simulink model "LC0419_nicholasye_fft"  (R2021b)
settings: Solver=VariableStepAuto  StartTime=0.0  StopTime=0.4  MaxStep=1e-4  RelTol=1e-3
libraries: spsSeriesRLCBranchLib x5, spsCurrentMeasurementLib x2, spsVoltageMeasurementLib x2, spsControlledVoltageSourceLib x1, spsGroundLib x1, spsTriangleGeneratorLib x1, spspowerguiLib x1
settings Model: Creator=98038  LastModifiedBy=NicholasYe
settings SolverCC: AlgebraicLoopSolver=TrustRegion
settings DataIOCC: ReturnWorkspaceOutputs=off
settings DebuggingCC: SFMachineParentedDataDiag=warning  ArithmeticOperatorsInVariantConditions=warning
settings SFSimCC: SimUseLocalCustomCode=off  CustomCodeUndefinedFunction=UseInterfaceOnly
settings RTWCC: RTWUseLocalCustomCode=off

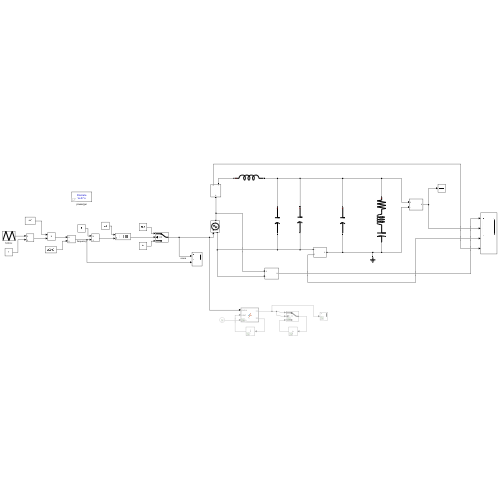
[thumbnail: Simulink's stored preview of the top-level diagram]
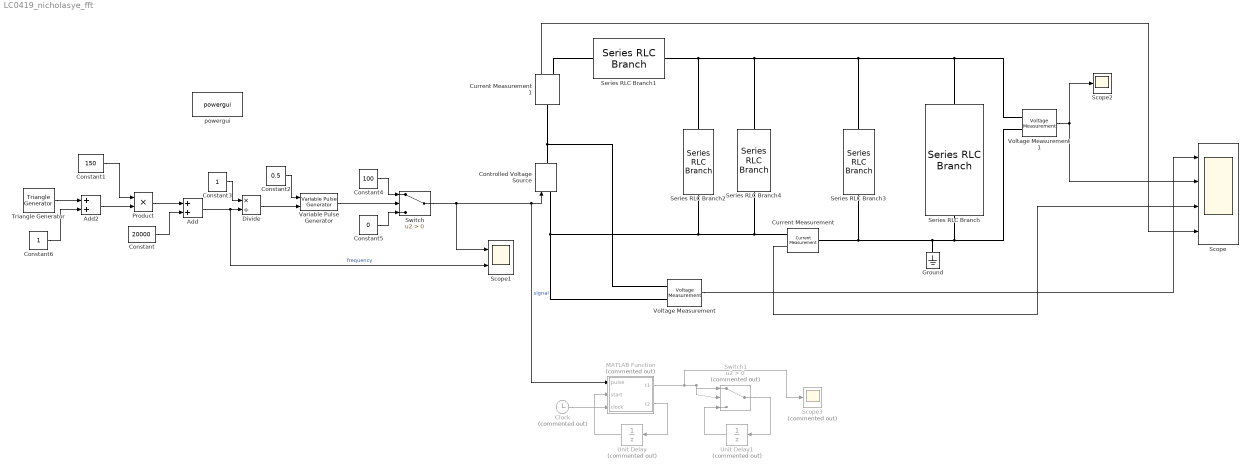
== system LC0419_nicholasye_fft ==
  Add : Sum
  Add2 : Sum
  Clock : Clock  Commented=on
  Constant : Constant  Value=20000
  Constant1 : Constant  Value=150
  Constant2 : Constant  Value=0.5
  Constant3 : Constant
  Constant4 : Constant  Value=100
  Constant5 : Constant  Value=0
  Constant6 : Constant
  Controlled Voltage Source : spsControlledVoltageSourceLib/Controlled Voltage Source  Initialize=off  Source_Type=AC  Amplitude=1  Phase=0  Frequency=20000  Measurements=Voltage
  Current Measurement : spsCurrentMeasurementLib/Current Measurement  PhasorSimulation=off  OutputType=Complex  PSBequivalent=0
  Current Measurement1 : spsCurrentMeasurementLib/Current Measurement  PhasorSimulation=off  OutputType=Complex  PSBequivalent=0
  Divide : Product  Inputs=*/
  Ground : spsGroundLib/Ground  LConnTagsString=a
  MATLAB Function : MATLAB Function  Commented=on  TreatAsAtomicUnit=on
  Product : Product
  Scope : Scope  NumInputPorts=4
  Scope1 : Scope  NumInputPorts=2
  Scope2 : Scope
  Scope3 : Scope  Commented=on
  Series RLC Branch : spsSeriesRLCBranchLib/Series RLC Branch  LConnTagsString=__new0  RConnTagsString=__new0  BranchType=RLC  Resistance=124.09  Inductance=1.463  SetiL0=off  InitialCurrent=0  Capacitance=42.528e-12  Setx0=off  InitialVoltage=0  Measurements=None
  Series RLC Branch1 : spsSeriesRLCBranchLib/Series RLC Branch  LConnTagsString=__new0  RConnTagsString=__new0  BranchType=L  Resistance=0  Inductance=0.00134  SetiL0=off  InitialCurrent=0  Capacitance=inf  Setx0=off  InitialVoltage=0  Measurements=None
  Series RLC Branch2 : spsSeriesRLCBranchLib/Series RLC Branch  LConnTagsString=__new0  RConnTagsString=__new0  BranchType=C  Resistance=0  Inductance=inf  SetiL0=off  InitialCurrent=0  Capacitance=6.8e-9  Setx0=off  InitialVoltage=0  Measurements=None
  Series RLC Branch3 : spsSeriesRLCBranchLib/Series RLC Branch  LConnTagsString=__new0  RConnTagsString=__new0  BranchType=C  Resistance=0  Inductance=inf  SetiL0=off  InitialCurrent=0  Capacitance=12.023e-9  Setx0=off  InitialVoltage=0  Measurements=None
  Series RLC Branch4 : spsSeriesRLCBranchLib/Series RLC Branch  LConnTagsString=__new0  RConnTagsString=__new0  BranchType=C  Resistance=0  Inductance=inf  SetiL0=off  InitialCurrent=0  Capacitance=6.8e-9  Setx0=off  InitialVoltage=0  Measurements=None
  Switch : Switch  Criteria=u2 > Threshold
  Switch1 : Switch  Commented=on  Criteria=u2 > Threshold
  Triangle Generator : spsTriangleGeneratorLib/Triangle Generator  Freq=500  Phase=0  Ts=0
      settings: AttributesFormatString=%<Freq>Hz
  Unit Delay : UnitDelay  Commented=on  SampleTime=-1  HasFrameUpgradeWarning=on
  Unit Delay1 : UnitDelay  Commented=on  SampleTime=-1  HasFrameUpgradeWarning=on
  Variable Pulse Generator : VariablePulseGenerator  SampleTime=0.1
  Voltage Measurement : spsVoltageMeasurementLib/Voltage Measurement  PhasorSimulation=off  OutputType=Complex  PSBequivalent=0
  Voltage Measurement1 : spsVoltageMeasurementLib/Voltage Measurement  PhasorSimulation=off  OutputType=Complex  PSBequivalent=0
  powergui : spspowerguiLib/powergui  Priority=1  SimulationMode=Discrete  SampleTime=1e-7  frequency=60  Iterations=50  frequencyindice=0  Pbase=100e6  ErrMax=1e-4  UnitsV=kV  UnitsW=MW  buscounter=0  FunctionMessages=off  echomessages=off  EnableUseOfTLC=off  CurrentSourceSwitches=off  DisableSnubberDevices=off  DisableRonSwitches=off  DisableVfSwitches=off  DisplayEquations=off  AutomaticDiscreteSolvers=off  SolverType=Tustin/Backward Euler (TBE)  Interpol=off  ExternalGateDelay=off  methode=off  Ts=100  x0status=blocks  SPID=on  SwTol=0  HookPort=off  NonlinearTolerance=1e-4  nMaxIteration=100  ContinueOnMaxIteration=off  RestoreLinks=warning  ResistiveCurrentMeasurement=off  Frange=[0:2:500]  Ylog=off  Xlog=on  ShowGrid=off  save=off  variable=ZData  structure=0  ZoomFFT=off  StartTime=0.0  cycles=1  DisplayStyle=1  fundamental=60  FreqAxis=off  MaxFrequency=1000  frequencyindicesteady=1  RmsSteady=1  display=off
  wires:
  Constant/1 -> Add/2
  Add2/1 -> Product/2
  Constant6/1 -> Add2/2
  Triangle Generator/1 -> Add2/1
  Constant3/1 -> Divide/1
  Constant2/1 -> Variable Pulse Generator/1
  Add/1 -> Scope1/2, Divide/2  "frequency"
  Constant1/1 -> Product/1
  Divide/1 -> Variable Pulse Generator/2
  Current Measurement1/1 -> Scope/4
  Current Measurement/1 -> Scope/3
  Voltage Measurement/1 -> Scope/1
  Voltage Measurement1/1 -> Scope2/1, Scope/2
  Variable Pulse Generator/1 -> Switch/2
  Constant4/1 -> Switch/1
  Constant5/1 -> Switch/3
  Switch/1 -> MATLAB Function/1(pulse), Controlled Voltage Source/1, Scope1/1  "signal"
  Product/1 -> Add/1
  Clock/1 -> MATLAB Function/3(clock)
  MATLAB Function/2(t2) -> Unit Delay/1
  Unit Delay/1 -> MATLAB Function/2(start)
  MATLAB Function/1(t1) -> Scope3/1, Switch1/2, Switch1/1
  Switch1/1 -> Unit Delay1/1
  Unit Delay1/1 -> Switch1/3
  connections:
  Controlled Voltage Source/LConn1 -- Series RLC Branch4/RConn1 -- Current Measurement/RConn1 -- Series RLC Branch2/RConn1 -- Voltage Measurement/LConn2
  Series RLC Branch4/LConn1 -- Series RLC Branch2/LConn1 -- Series RLC Branch1/RConn1 -- Series RLC Branch/LConn1 -- Voltage Measurement1/LConn1 -- Series RLC Branch3/LConn1
  Voltage Measurement/LConn1 -- Current Measurement1/LConn1 -- Controlled Voltage Source/RConn1
  Voltage Measurement1/LConn2 -- Current Measurement/LConn1 -- Series RLC Branch3/RConn1 -- Ground/LConn1 -- Series RLC Branch/RConn1
  Series RLC Branch1/LConn1 -- Current Measurement1/RConn1

== matlab function LC0419_nicholasye_fft/MATLAB Function ==
  data: t1 output; pulse input; start input; t2 output; clock input
function [t1, t2] = fcn(pulse, start, clock)

temp = start;

if pulse > 0
    t1 = clock - temp;
else
    t1 = 0;
end

t2 = clock;
